simulink model "TST_EngDem_TrqLimCoord"  (R2016b)
settings: Solver=FixedStepDiscrete  StartTime=0.0  StopTime=0  FixedStep=sampleTime  RelTol=1e-3
values from neighbouring files (symbols this model uses):
  testCase = 1    [initTST_EngDem_TrqLimCoord_001.m]    (also in initTST_EngDem_TrqLimCoord_002.m = 2; initTST_EngDem_TrqLimCoord_003.m = 3; initTST_EngDem_TrqLimCoord_004.m = 4)
libraries: simulink x33, UnitTest_Lib x28
(part 2 of 2)

== system TST_EngDem_TrqLimCoord/simulationInput/testSignals_R004 ==
  BC : BusCreator  Inputs=22
  spec_ASMod_dvolPFltEG : FromWorkspace  VariableName=testSig_ASMod_dvolPFltEG  Interpolate=off  OutputAfterFinalValue=Holding final value
  spec_CoETS_trqNTCLim : FromWorkspace  VariableName=testSig_CoETS_trqNTCLim  Interpolate=off  OutputAfterFinalValue=Holding final value
  spec_CoVeh_trqPrfmLimDes : FromWorkspace  VariableName=testSig_CoVeh_trqPrfmLimDes  Interpolate=off  OutputAfterFinalValue=Holding final value
  spec_DSM_bEngDemTrqLimErr1 : FromWorkspace  VariableName=testSig_DSM_bEngDemTrqLimErr1  Interpolate=off  OutputAfterFinalValue=Holding final value
  spec_DSM_bEngDemTrqLimErr2 : FromWorkspace  VariableName=testSig_DSM_bEngDemTrqLimErr2  Interpolate=off  OutputAfterFinalValue=Holding final value
  spec_DSM_bEngDemTrqLimErr3 : FromWorkspace  VariableName=testSig_DSM_bEngDemTrqLimErr3  Interpolate=off  OutputAfterFinalValue=Holding final value
  spec_DSM_bEngDemTrqLimErr4 : FromWorkspace  VariableName=testSig_DSM_bEngDemTrqLimErr4  Interpolate=off  OutputAfterFinalValue=Holding final value
  spec_EngDem_facAdj : FromWorkspace  VariableName=testSig_EngDem_facAdj  Interpolate=off  OutputAfterFinalValue=Holding final value
  spec_EngDem_stErr_mp : FromWorkspace  VariableName=testSig_EngDem_stErr_mp  Interpolate=off  OutputAfterFinalValue=Holding final value
  spec_EngDem_trqInrLim : FromWorkspace  VariableName=testSig_EngDem_trqInrLim  Interpolate=off  OutputAfterFinalValue=Holding final value
  spec_EngDem_trqInrLimLead : FromWorkspace  VariableName=testSig_EngDem_trqInrLimLead  Interpolate=off  OutputAfterFinalValue=Holding final value
  spec_EngDem_trqInrLimSlow : FromWorkspace  VariableName=testSig_EngDem_trqInrLimSlow  Interpolate=off  OutputAfterFinalValue=Holding final value
  spec_EngDem_trqLimErr : FromWorkspace  VariableName=testSig_EngDem_trqLimErr  Interpolate=off  OutputAfterFinalValue=Holding final value
  spec_EngDem_trqLimPDiff : FromWorkspace  VariableName=testSig_EngDem_trqLimPDiff  Interpolate=off  OutputAfterFinalValue=Holding final value
  spec_EngPrt_trqLim : FromWorkspace  VariableName=testSig_EngPrt_trqLim  Interpolate=off  OutputAfterFinalValue=Holding final value
  spec_EngReq_trqInrLimSmk : FromWorkspace  VariableName=testSig_EngReq_trqInrLimSmk  Interpolate=off  OutputAfterFinalValue=Holding final value
  spec_EngReq_trqLim : FromWorkspace  VariableName=testSig_EngReq_trqLim  Interpolate=off  OutputAfterFinalValue=Holding final value
  spec_Epm_nEng : FromWorkspace  VariableName=testSig_Epm_nEng  Interpolate=off  OutputAfterFinalValue=Holding final value
  spec_GlbDa_stTrqDem : FromWorkspace  VariableName=testSig_GlbDa_stTrqDem  Interpolate=off  OutputAfterFinalValue=Holding final value
  spec_PFltLd_resFlw : FromWorkspace  VariableName=testSig_PFltLd_resFlw  Interpolate=off  OutputAfterFinalValue=Holding final value
  spec_TCPrt_trqInrBstPrtLim : FromWorkspace  VariableName=testSig_TCPrt_trqInrBstPrtLim  Interpolate=off  OutputAfterFinalValue=Holding final value
  spec_Tra_trqDblClthEngMax : FromWorkspace  VariableName=testSig_Tra_trqDblClthEngMax  Interpolate=off  OutputAfterFinalValue=Holding final value
  testSignals : Outport
  wires:
  BC/1 -> testSignals/1
  spec_Epm_nEng/1 -> BC/1  "testSig_Epm_nEng"
  spec_Tra_trqDblClthEngMax/1 -> BC/2  "testSig_Tra_trqDblClthEngMax"
  spec_TCPrt_trqInrBstPrtLim/1 -> BC/3  "testSig_TCPrt_trqInrBstPrtLim"
  spec_EngReq_trqLim/1 -> BC/4  "testSig_EngReq_trqLim"
  spec_GlbDa_stTrqDem/1 -> BC/5  "testSig_GlbDa_stTrqDem"
  spec_EngReq_trqInrLimSmk/1 -> BC/6  "testSig_EngReq_trqInrLimSmk"
  spec_EngPrt_trqLim/1 -> BC/7  "testSig_EngPrt_trqLim"
  spec_DSM_bEngDemTrqLimErr1/1 -> BC/8  "testSig_DSM_bEngDemTrqLimErr1"
  spec_DSM_bEngDemTrqLimErr2/1 -> BC/9  "testSig_DSM_bEngDemTrqLimErr2"
  spec_DSM_bEngDemTrqLimErr3/1 -> BC/10  "testSig_DSM_bEngDemTrqLimErr3"
  spec_DSM_bEngDemTrqLimErr4/1 -> BC/11  "testSig_DSM_bEngDemTrqLimErr4"
  spec_ASMod_dvolPFltEG/1 -> BC/12  "testSig_ASMod_dvolPFltEG"
  spec_PFltLd_resFlw/1 -> BC/13  "testSig_PFltLd_resFlw"
  spec_CoETS_trqNTCLim/1 -> BC/14  "testSig_CoETS_trqNTCLim"
  spec_CoVeh_trqPrfmLimDes/1 -> BC/15  "testSig_CoVeh_trqPrfmLimDes"
  spec_EngDem_trqLimErr/1 -> BC/16  "testSig_EngDem_trqLimErr"
  spec_EngDem_trqLimPDiff/1 -> BC/17  "testSig_EngDem_trqLimPDiff"
  spec_EngDem_trqInrLim/1 -> BC/18  "testSig_EngDem_trqInrLim"
  spec_EngDem_stErr_mp/1 -> BC/19  "testSig_EngDem_stErr_mp"
  spec_EngDem_facAdj/1 -> BC/20  "testSig_EngDem_facAdj"
  spec_EngDem_trqInrLimLead/1 -> BC/21  "testSig_EngDem_trqInrLimLead"
  spec_EngDem_trqInrLimSlow/1 -> BC/22  "testSig_EngDem_trqInrLimSlow"

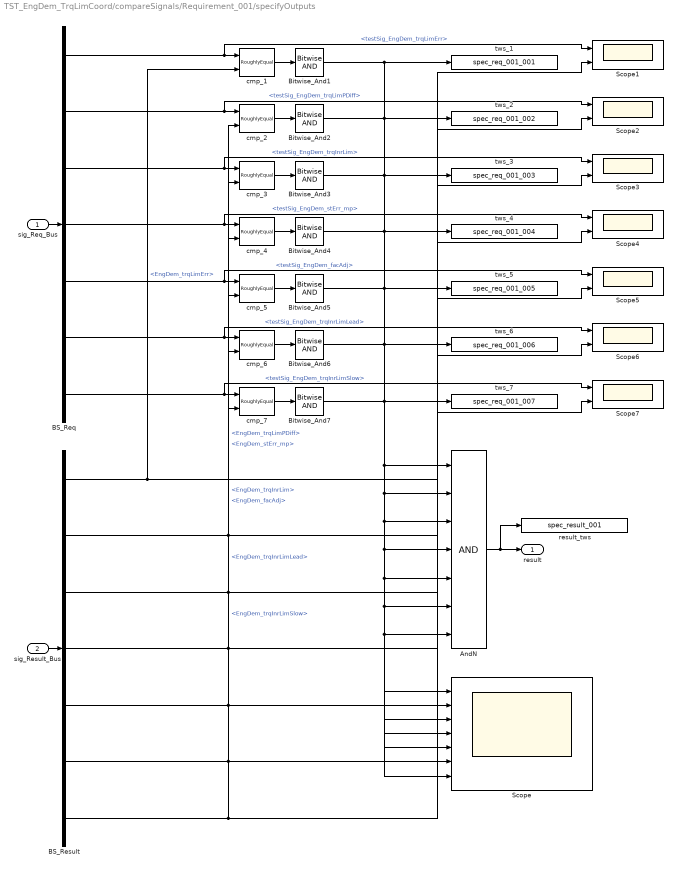
== system TST_EngDem_TrqLimCoord/compareSignals/Requirement_001/specifyOutputs ==
  sig_Req_Bus : Inport
  sig_Result_Bus : Inport  Port=2
  AndN : Logic  Inputs=7
  BS_Req : BusSelector  OutputSignals=testSig_EngDem_trqLimErr,testSig_EngDem_trqLimPDiff,testSig_EngDem_trqInrLim,testSig_EngDem_stErr_mp,testSig_EngDem_facAdj,testSig_EngDem_trqInrLimLead,testSig_EngDem_trqInrLimSlow
  BS_Result : BusSelector  OutputSignals=EngDem_trqLimErr,EngDem_trqLimPDiff,EngDem_trqInrLim,EngDem_stErr_mp,EngDem_facAdj,EngDem_trqInrLimLead,EngDem_trqInrLimSlow
  Bitwise_And{1..7} (7 alike) : simulink/Logic and Bit Operations/Bitwise Operator  logicop=AND  UseBitMask=off  BitMask=bin2dec('11011001')  BitMaskRealWorld=Stored Integer
  Scope : Scope  NumInputPorts=7
  Scope{1..7} (7 alike) : Scope  NumInputPorts=2
  cmp_1 : UnitTest_Lib/RoughlyEqual  slope=1
  cmp_{2..7} (6 alike) : UnitTest_Lib/RoughlyEqual  slope=0.1
  result_tws : ToWorkspace  VariableName=spec_result_001
  tws_1 : ToWorkspace  VariableName=spec_req_001_001
  tws_2 : ToWorkspace  VariableName=spec_req_001_002
  tws_3 : ToWorkspace  VariableName=spec_req_001_003
  tws_4 : ToWorkspace  VariableName=spec_req_001_004
  tws_5 : ToWorkspace  VariableName=spec_req_001_005
  tws_6 : ToWorkspace  VariableName=spec_req_001_006
  tws_7 : ToWorkspace  VariableName=spec_req_001_007
  result : Outport
  wires:
  sig_Req_Bus/1 -> BS_Req/1
  sig_Result_Bus/1 -> BS_Result/1
  AndN/1 -> result/1, result_tws/1
  BS_Req/1 -> cmp_1/1, Scope1/1  "<testSig_EngDem_trqLimErr>"
  BS_Result/1 -> cmp_1/2, Scope1/2  "<EngDem_trqLimErr>"
  cmp_1/1 -> Bitwise_And1/1
  Bitwise_And1/1 -> AndN/1, Scope/1, tws_1/1
  BS_Req/2 -> cmp_2/1, Scope2/1  "<testSig_EngDem_trqLimPDiff>"
  BS_Result/2 -> cmp_2/2, Scope2/2  "<EngDem_trqLimPDiff>"
  cmp_2/1 -> Bitwise_And2/1
  Bitwise_And2/1 -> AndN/2, Scope/2, tws_2/1
  BS_Req/3 -> cmp_3/1, Scope3/1  "<testSig_EngDem_trqInrLim>"
  BS_Result/3 -> cmp_3/2, Scope3/2  "<EngDem_trqInrLim>"
  cmp_3/1 -> Bitwise_And3/1
  Bitwise_And3/1 -> AndN/3, Scope/3, tws_3/1
  BS_Req/4 -> cmp_4/1, Scope4/1  "<testSig_EngDem_stErr_mp>"
  BS_Result/4 -> cmp_4/2, Scope4/2  "<EngDem_stErr_mp>"
  cmp_4/1 -> Bitwise_And4/1
  Bitwise_And4/1 -> AndN/4, Scope/4, tws_4/1
  BS_Req/5 -> cmp_5/1, Scope5/1  "<testSig_EngDem_facAdj>"
  BS_Result/5 -> cmp_5/2, Scope5/2  "<EngDem_facAdj>"
  cmp_5/1 -> Bitwise_And5/1
  Bitwise_And5/1 -> AndN/5, Scope/5, tws_5/1
  BS_Req/6 -> cmp_6/1, Scope6/1  "<testSig_EngDem_trqInrLimLead>"
  BS_Result/6 -> cmp_6/2, Scope6/2  "<EngDem_trqInrLimLead>"
  cmp_6/1 -> Bitwise_And6/1
  Bitwise_And6/1 -> AndN/6, Scope/6, tws_6/1
  BS_Req/7 -> cmp_7/1, Scope7/1  "<testSig_EngDem_trqInrLimSlow>"
  BS_Result/7 -> cmp_7/2, Scope7/2  "<EngDem_trqInrLimSlow>"
  cmp_7/1 -> Bitwise_And7/1
  Bitwise_And7/1 -> AndN/7, Scope/7, tws_7/1

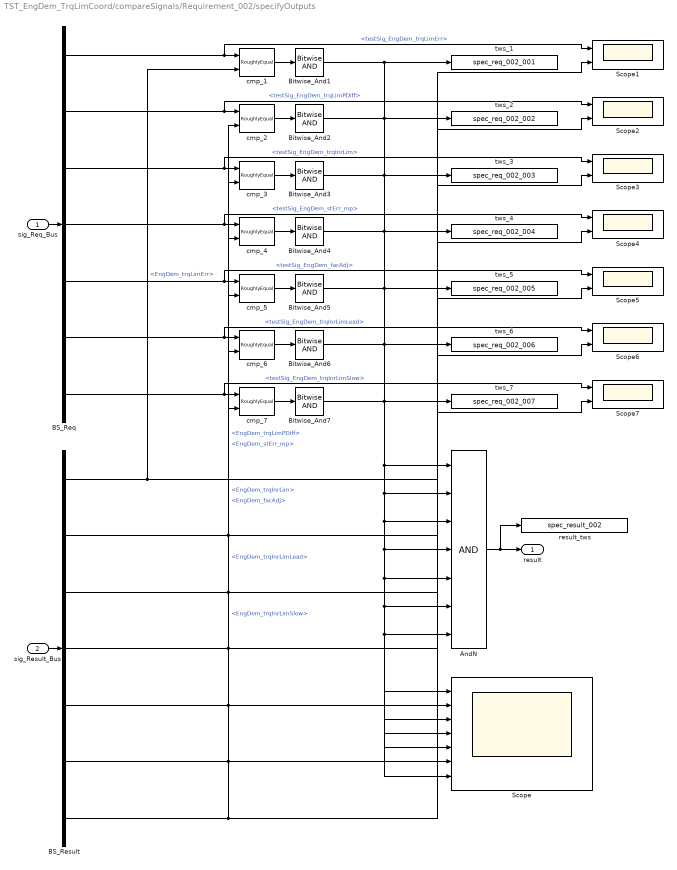
== system TST_EngDem_TrqLimCoord/compareSignals/Requirement_002/specifyOutputs ==
  sig_Req_Bus : Inport
  sig_Result_Bus : Inport  Port=2
  AndN : Logic  Inputs=7
  BS_Req : BusSelector  OutputSignals=testSig_EngDem_trqLimErr,testSig_EngDem_trqLimPDiff,testSig_EngDem_trqInrLim,testSig_EngDem_stErr_mp,testSig_EngDem_facAdj,testSig_EngDem_trqInrLimLead,testSig_EngDem_trqInrLimSlow
  BS_Result : BusSelector  OutputSignals=EngDem_trqLimErr,EngDem_trqLimPDiff,EngDem_trqInrLim,EngDem_stErr_mp,EngDem_facAdj,EngDem_trqInrLimLead,EngDem_trqInrLimSlow
  Bitwise_And{1..7} (7 alike) : simulink/Logic and Bit Operations/Bitwise Operator  logicop=AND  UseBitMask=off  BitMask=bin2dec('11011001')  BitMaskRealWorld=Stored Integer
  Scope : Scope  NumInputPorts=7
  Scope{1..7} (7 alike) : Scope  NumInputPorts=2
  cmp_{1,3,6..7} (4 alike) : UnitTest_Lib/RoughlyEqual  slope=1
  cmp_2 : UnitTest_Lib/RoughlyEqual  slope=0.1
  cmp_4 : UnitTest_Lib/RoughlyEqual  slope=0.1
  cmp_5 : UnitTest_Lib/RoughlyEqual  slope=0.1
  result_tws : ToWorkspace  VariableName=spec_result_002
  tws_1 : ToWorkspace  VariableName=spec_req_002_001
  tws_2 : ToWorkspace  VariableName=spec_req_002_002
  tws_3 : ToWorkspace  VariableName=spec_req_002_003
  tws_4 : ToWorkspace  VariableName=spec_req_002_004
  tws_5 : ToWorkspace  VariableName=spec_req_002_005
  tws_6 : ToWorkspace  VariableName=spec_req_002_006
  tws_7 : ToWorkspace  VariableName=spec_req_002_007
  result : Outport
  wires:
  sig_Req_Bus/1 -> BS_Req/1
  sig_Result_Bus/1 -> BS_Result/1
  AndN/1 -> result/1, result_tws/1
  BS_Req/1 -> cmp_1/1, Scope1/1  "<testSig_EngDem_trqLimErr>"
  BS_Result/1 -> cmp_1/2, Scope1/2  "<EngDem_trqLimErr>"
  cmp_1/1 -> Bitwise_And1/1
  Bitwise_And1/1 -> AndN/1, Scope/1, tws_1/1
  BS_Req/2 -> cmp_2/1, Scope2/1  "<testSig_EngDem_trqLimPDiff>"
  BS_Result/2 -> cmp_2/2, Scope2/2  "<EngDem_trqLimPDiff>"
  cmp_2/1 -> Bitwise_And2/1
  Bitwise_And2/1 -> AndN/2, Scope/2, tws_2/1
  BS_Req/3 -> cmp_3/1, Scope3/1  "<testSig_EngDem_trqInrLim>"
  BS_Result/3 -> cmp_3/2, Scope3/2  "<EngDem_trqInrLim>"
  cmp_3/1 -> Bitwise_And3/1
  Bitwise_And3/1 -> AndN/3, Scope/3, tws_3/1
  BS_Req/4 -> cmp_4/1, Scope4/1  "<testSig_EngDem_stErr_mp>"
  BS_Result/4 -> cmp_4/2, Scope4/2  "<EngDem_stErr_mp>"
  cmp_4/1 -> Bitwise_And4/1
  Bitwise_And4/1 -> AndN/4, Scope/4, tws_4/1
  BS_Req/5 -> cmp_5/1, Scope5/1  "<testSig_EngDem_facAdj>"
  BS_Result/5 -> cmp_5/2, Scope5/2  "<EngDem_facAdj>"
  cmp_5/1 -> Bitwise_And5/1
  Bitwise_And5/1 -> AndN/5, Scope/5, tws_5/1
  BS_Req/6 -> cmp_6/1, Scope6/1  "<testSig_EngDem_trqInrLimLead>"
  BS_Result/6 -> cmp_6/2, Scope6/2  "<EngDem_trqInrLimLead>"
  cmp_6/1 -> Bitwise_And6/1
  Bitwise_And6/1 -> AndN/6, Scope/6, tws_6/1
  BS_Req/7 -> cmp_7/1, Scope7/1  "<testSig_EngDem_trqInrLimSlow>"
  BS_Result/7 -> cmp_7/2, Scope7/2  "<EngDem_trqInrLimSlow>"
  cmp_7/1 -> Bitwise_And7/1
  Bitwise_And7/1 -> AndN/7, Scope/7, tws_7/1

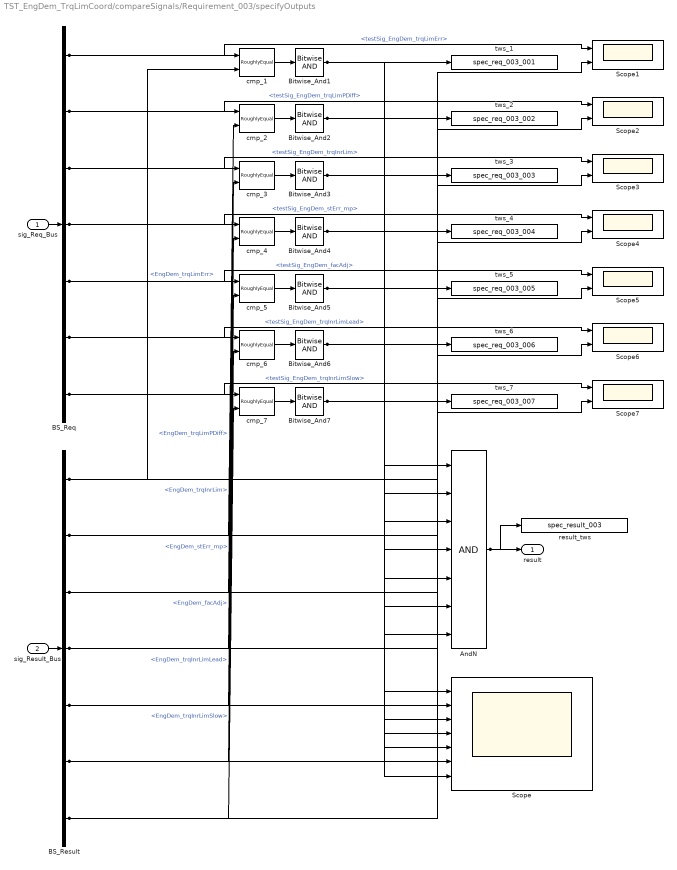
== system TST_EngDem_TrqLimCoord/compareSignals/Requirement_003/specifyOutputs ==
  sig_Req_Bus : Inport
  sig_Result_Bus : Inport  Port=2
  AndN : Logic  Inputs=7
  BS_Req : BusSelector  OutputSignals=testSig_EngDem_trqLimErr,testSig_EngDem_trqLimPDiff,testSig_EngDem_trqInrLim,testSig_EngDem_stErr_mp,testSig_EngDem_facAdj,testSig_EngDem_trqInrLimLead,testSig_EngDem_trqInrLimSlow
  BS_Result : BusSelector  OutputSignals=EngDem_trqLimErr,EngDem_trqLimPDiff,EngDem_trqInrLim,EngDem_stErr_mp,EngDem_facAdj,EngDem_trqInrLimLead,EngDem_trqInrLimSlow
  Bitwise_And{1..7} (7 alike) : simulink/Logic and Bit Operations/Bitwise Operator  logicop=AND  UseBitMask=off  BitMask=bin2dec('11011001')  BitMaskRealWorld=Stored Integer
  Scope : Scope  NumInputPorts=7
  Scope{1..7} (7 alike) : Scope  NumInputPorts=2
  cmp_{1..7} (7 alike) : UnitTest_Lib/RoughlyEqual  slope=0.1
  result_tws : ToWorkspace  VariableName=spec_result_003
  tws_1 : ToWorkspace  VariableName=spec_req_003_001
  tws_2 : ToWorkspace  VariableName=spec_req_003_002
  tws_3 : ToWorkspace  VariableName=spec_req_003_003
  tws_4 : ToWorkspace  VariableName=spec_req_003_004
  tws_5 : ToWorkspace  VariableName=spec_req_003_005
  tws_6 : ToWorkspace  VariableName=spec_req_003_006
  tws_7 : ToWorkspace  VariableName=spec_req_003_007
  result : Outport
  wires:
  sig_Req_Bus/1 -> BS_Req/1
  sig_Result_Bus/1 -> BS_Result/1
  AndN/1 -> result/1, result_tws/1
  BS_Req/1 -> cmp_1/1, Scope1/1  "<testSig_EngDem_trqLimErr>"
  BS_Result/1 -> cmp_1/2, Scope1/2  "<EngDem_trqLimErr>"
  cmp_1/1 -> Bitwise_And1/1
  Bitwise_And1/1 -> tws_1/1, AndN/1, Scope/1
  BS_Req/2 -> cmp_2/1, Scope2/1  "<testSig_EngDem_trqLimPDiff>"
  BS_Result/2 -> cmp_2/2, Scope2/2  "<EngDem_trqLimPDiff>"
  cmp_2/1 -> Bitwise_And2/1
  Bitwise_And2/1 -> tws_2/1, AndN/2, Scope/2
  BS_Req/3 -> cmp_3/1, Scope3/1  "<testSig_EngDem_trqInrLim>"
  BS_Result/3 -> cmp_3/2, Scope3/2  "<EngDem_trqInrLim>"
  cmp_3/1 -> Bitwise_And3/1
  Bitwise_And3/1 -> tws_3/1, AndN/3, Scope/3
  BS_Req/4 -> cmp_4/1, Scope4/1  "<testSig_EngDem_stErr_mp>"
  BS_Result/4 -> cmp_4/2, Scope4/2  "<EngDem_stErr_mp>"
  cmp_4/1 -> Bitwise_And4/1
  Bitwise_And4/1 -> tws_4/1, AndN/4, Scope/4
  BS_Req/5 -> cmp_5/1, Scope5/1  "<testSig_EngDem_facAdj>"
  BS_Result/5 -> cmp_5/2, Scope5/2  "<EngDem_facAdj>"
  cmp_5/1 -> Bitwise_And5/1
  Bitwise_And5/1 -> tws_5/1, AndN/5, Scope/5
  BS_Req/6 -> cmp_6/1, Scope6/1  "<testSig_EngDem_trqInrLimLead>"
  BS_Result/6 -> cmp_6/2, Scope6/2  "<EngDem_trqInrLimLead>"
  cmp_6/1 -> Bitwise_And6/1
  Bitwise_And6/1 -> tws_6/1, AndN/6, Scope/6
  BS_Req/7 -> cmp_7/1, Scope7/1  "<testSig_EngDem_trqInrLimSlow>"
  BS_Result/7 -> cmp_7/2, Scope7/2  "<EngDem_trqInrLimSlow>"
  cmp_7/1 -> Bitwise_And7/1
  Bitwise_And7/1 -> tws_7/1, AndN/7, Scope/7

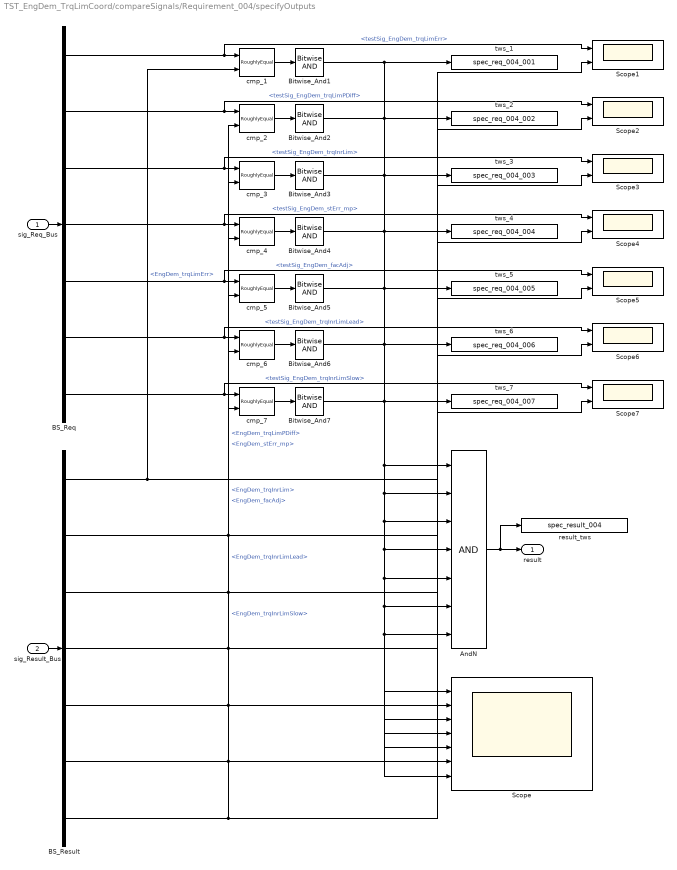
== system TST_EngDem_TrqLimCoord/compareSignals/Requirement_004/specifyOutputs ==
  sig_Req_Bus : Inport
  sig_Result_Bus : Inport  Port=2
  AndN : Logic  Inputs=7
  BS_Req : BusSelector  OutputSignals=testSig_EngDem_trqLimErr,testSig_EngDem_trqLimPDiff,testSig_EngDem_trqInrLim,testSig_EngDem_stErr_mp,testSig_EngDem_facAdj,testSig_EngDem_trqInrLimLead,testSig_EngDem_trqInrLimSlow
  BS_Result : BusSelector  OutputSignals=EngDem_trqLimErr,EngDem_trqLimPDiff,EngDem_trqInrLim,EngDem_stErr_mp,EngDem_facAdj,EngDem_trqInrLimLead,EngDem_trqInrLimSlow
  Bitwise_And{1..7} (7 alike) : simulink/Logic and Bit Operations/Bitwise Operator  logicop=AND  UseBitMask=off  BitMask=bin2dec('11011001')  BitMaskRealWorld=Stored Integer
  Scope : Scope  NumInputPorts=7
  Scope{1..7} (7 alike) : Scope  NumInputPorts=2
  cmp_{1,3,6..7} (4 alike) : UnitTest_Lib/RoughlyEqual  slope=1
  cmp_2 : UnitTest_Lib/RoughlyEqual  slope=0.1
  cmp_4 : UnitTest_Lib/RoughlyEqual  slope=0.1
  cmp_5 : UnitTest_Lib/RoughlyEqual  slope=0.1
  result_tws : ToWorkspace  VariableName=spec_result_004
  tws_1 : ToWorkspace  VariableName=spec_req_004_001
  tws_2 : ToWorkspace  VariableName=spec_req_004_002
  tws_3 : ToWorkspace  VariableName=spec_req_004_003
  tws_4 : ToWorkspace  VariableName=spec_req_004_004
  tws_5 : ToWorkspace  VariableName=spec_req_004_005
  tws_6 : ToWorkspace  VariableName=spec_req_004_006
  tws_7 : ToWorkspace  VariableName=spec_req_004_007
  result : Outport
  wires:
  sig_Req_Bus/1 -> BS_Req/1
  sig_Result_Bus/1 -> BS_Result/1
  AndN/1 -> result/1, result_tws/1
  BS_Req/1 -> cmp_1/1, Scope1/1  "<testSig_EngDem_trqLimErr>"
  BS_Result/1 -> cmp_1/2, Scope1/2  "<EngDem_trqLimErr>"
  cmp_1/1 -> Bitwise_And1/1
  Bitwise_And1/1 -> AndN/1, Scope/1, tws_1/1
  BS_Req/2 -> cmp_2/1, Scope2/1  "<testSig_EngDem_trqLimPDiff>"
  BS_Result/2 -> cmp_2/2, Scope2/2  "<EngDem_trqLimPDiff>"
  cmp_2/1 -> Bitwise_And2/1
  Bitwise_And2/1 -> AndN/2, Scope/2, tws_2/1
  BS_Req/3 -> cmp_3/1, Scope3/1  "<testSig_EngDem_trqInrLim>"
  BS_Result/3 -> cmp_3/2, Scope3/2  "<EngDem_trqInrLim>"
  cmp_3/1 -> Bitwise_And3/1
  Bitwise_And3/1 -> AndN/3, Scope/3, tws_3/1
  BS_Req/4 -> cmp_4/1, Scope4/1  "<testSig_EngDem_stErr_mp>"
  BS_Result/4 -> cmp_4/2, Scope4/2  "<EngDem_stErr_mp>"
  cmp_4/1 -> Bitwise_And4/1
  Bitwise_And4/1 -> AndN/4, Scope/4, tws_4/1
  BS_Req/5 -> cmp_5/1, Scope5/1  "<testSig_EngDem_facAdj>"
  BS_Result/5 -> cmp_5/2, Scope5/2  "<EngDem_facAdj>"
  cmp_5/1 -> Bitwise_And5/1
  Bitwise_And5/1 -> AndN/5, Scope/5, tws_5/1
  BS_Req/6 -> cmp_6/1, Scope6/1  "<testSig_EngDem_trqInrLimLead>"
  BS_Result/6 -> cmp_6/2, Scope6/2  "<EngDem_trqInrLimLead>"
  cmp_6/1 -> Bitwise_And6/1
  Bitwise_And6/1 -> AndN/6, Scope/6, tws_6/1
  BS_Req/7 -> cmp_7/1, Scope7/1  "<testSig_EngDem_trqInrLimSlow>"
  BS_Result/7 -> cmp_7/2, Scope7/2  "<EngDem_trqInrLimSlow>"
  cmp_7/1 -> Bitwise_And7/1
  Bitwise_And7/1 -> AndN/7, Scope/7, tws_7/1
